simulink model "simPractica14"  (R2020b)
settings: Solver=VariableStepAuto  StartTime=0.0  StopTime=2000  RelTol=1e-3
libraries: fuzblock x1
settings Model: Creator=COMETA  LastModifiedBy=COMETA

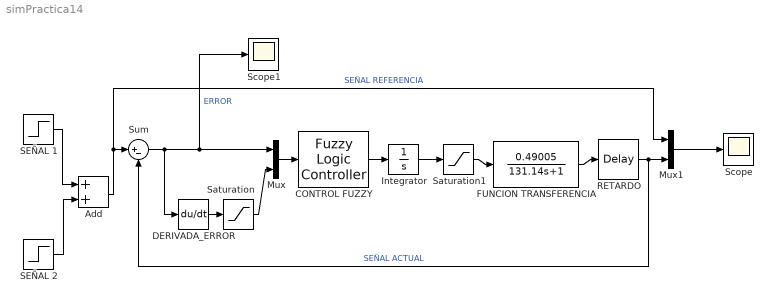
== system simPractica14 ==
  Add : Sum
  CONTROL FUZZY : fuzblock/Fuzzy Logic  Controller  FIS=demo12_Final  OutputSampleNumber=101  DataType=double  FuzzifiedInputs=off  RuleFiringStrengths=off  RuleOutputs=off  AggregatedOutputs=off  SimulateUsing=Interpreted execution  OutOfRangeInputValueMessage=warning  NoRuleFiredMessage=warning  EmptyOutputFuzzySetMessage=warning
  DERIVADA_ERROR : Derivative
  "FUNCION TRANSFERENCIA " : TransferFcn  Numerator=[0.49005]  Denominator=[131.14 1]
  Integrator : Integrator
  Mux : Mux  Inputs=2
  Mux1 : Mux  Inputs=2
  RETARDO : TransportDelay  DelayTime=30
  SEÑAL 1 : Step  Time=100  After=20  SampleTime=0
  SEÑAL 2 : Step  Time=1000  After=5  SampleTime=0
  Saturation : Saturate  UpperLimit=1  LowerLimit=-1
  Saturation1 : Saturate  UpperLimit=100  LowerLimit=0
  Scope : Scope
  Scope1 : Scope
  Sum : Sum  Inputs=|+-
  wires:
  DERIVADA_ERROR/1 -> Saturation/1
  Mux/1 -> CONTROL FUZZY/1
  CONTROL FUZZY/1 -> Integrator/1
  Saturation1/1 -> "FUNCION TRANSFERENCIA "/1
  "FUNCION TRANSFERENCIA "/1 -> RETARDO/1
  Saturation/1 -> Mux/2
  Integrator/1 -> Saturation1/1
  Sum/1 -> DERIVADA_ERROR/1, Scope1/1, Mux/1  "ERROR"
  SEÑAL 1/1 -> Add/1
  RETARDO/1 -> Mux1/2, Sum/2  "SEÑAL ACTUAL"
  Mux1/1 -> Scope/1
  SEÑAL 2/1 -> Add/2
  Add/1 -> Mux1/1, Sum/1  "SEÑAL REFERENCIA"
